simulink model "Model_14Bus_AC_DC_Microgrid"  (R2025a)
settings: Solver=ode23tb  StartTime=0.0  StopTime=0.1  MaxStep=1e-2  RelTol=1e-3
InitFcn:
  | Set_parameters_R2018
StopFcn:
  | Save_Data;
  | Graphics;
undefined symbols (not defined in the file): Clink, D1, Delta, dis1, dis10, dis11, dis12, dis13, dis14, dis2, dis3, dis4, dis5, dis6, dis7, dis8, dis9, Fc, Fnom, Hydride, Increment_MPPT, Ion, Ki_Ireg, Ki_VDCreg, Kp_Ireg, Kp_VDCreg, LimitL_Ireg, LimitL_VDCreg, Limits_MPPT, LimitU_Ireg, LimitU_VDCreg, Lithium, max_min, Metal, Nickel, P_Load_2, P_Load_3, Pnom, Pnom_T1, Pnom_T2, Pnom_T3, Pnom_xfo, Ql_Load_2, Ql_Load_3, R_Load_9, R_Load_DC, RL, Rl, RLff, Rls, sigbuilder_block, Ts, Ts_Control, Ts_Power, V1_LL_T3, Vf, Vfd, Vnom_dc, Vnom_DC, Vnom_Diesel ... (+5)
libraries: spsRMSLib x87, spsCurrentMeasurementLib x47, spsThreePhaseVIMeasurementLib x23, spsVoltageMeasurementLib x21, spsPowerLib x21, spsTHDLib x20, spsThreePhaseSeriesRLCBranchLib x20, spsSeriesRLCBranchLib x19, spsIGBTDiodeLib x14, spsThreePhaseBreakerLib x14, powerlib_extras x14, simulink x12
(part 8 of 9)

== system Model_14Bus_AC_DC_Microgrid/Bus_6 /PLL/Pll2 ==
  note: error
  note: d'
  note: Fundamental
  note: fase
      | total
  note: fase de la señal
  note: adelanta 90
  note: Este PLL calcula la fase respecto a una onda coseno
  señal : Inport
  w : Inport  Port=2
  Gain : Gain  Gain=-1  SaturateOnIntegerOverflow=on  OutDataTypeStr=Inherit: Same as input  ParamDataTypeStr=Inherit: Same as input
  Integrator : Integrator  InitialCondition=2*pi*60
  Integrator1 : Integrator  InitialCondition=2*pi*60
  Integrator2 : Integrator
  K : Gain  Gain=100  SaturateOnIntegerOverflow=on  OutDataTypeStr=Inherit: Same as input  ParamDataTypeStr=Inherit: Same as input
  Kp : Gain  Gain=10  SaturateOnIntegerOverflow=on  OutDataTypeStr=Inherit: Same as input  ParamDataTypeStr=Inherit: Same as input
  Kp1 : Gain  Gain=10  SaturateOnIntegerOverflow=on  OutDataTypeStr=Inherit: Same as input  ParamDataTypeStr=Inherit: Same as input
  Poduct : Product  SaturateOnIntegerOverflow=on  OutDataTypeStr=Inherit: Same as first input
  Poduct1 : Product  SaturateOnIntegerOverflow=on  OutDataTypeStr=Inherit: Same as first input
  Poduct2 : Product  SaturateOnIntegerOverflow=on  OutDataTypeStr=Inherit: Same as first input
  Sum : Sum  Inputs=|+-  SaturateOnIntegerOverflow=on
  Sum1 : Sum  SaturateOnIntegerOverflow=on
  Sum2 : Sum  Inputs=|-+  SaturateOnIntegerOverflow=on
  Trigonometric Function : Trigonometry
  Trigonometric Function1 : Trigonometry  Operator=cos
  f cos (rad) : Outport  VectorParamsAs1DForOutWhenUnconnected=off
  wires:
  Sum/1 -> Poduct/1, Poduct1/1
  Poduct/1 -> Kp/1
  Kp/1 -> Kp1/1
  Poduct2/1 -> Sum/2
  Trigonometric Function1/1 -> Poduct1/2, Poduct2/1
  Poduct1/1 -> K/1
  K/1 -> Integrator2/1
  Integrator2/1 -> Poduct2/2
  Integrator/1 -> Trigonometric Function/1, Sum2/2, Trigonometric Function1/1
  Integrator1/1 -> Sum2/1
  Sum2/1 -> f cos (rad)/1
  w/1 -> Sum1/1, Integrator1/1
  Kp1/1 -> Sum1/2
  Sum1/1 -> Integrator/1
  Trigonometric Function/1 -> Gain/1
  Gain/1 -> Poduct/2
  señal/1 -> Sum/1

== system Model_14Bus_AC_DC_Microgrid/Bus_6 /PLL/Pll3 ==
  note: error
  note: d'
  note: Fundamental
  note: fase
      | total
  note: fase de la señal
  note: adelanta 90
  note: Este PLL calcula la fase respecto a una onda coseno
  señal : Inport
  w : Inport  Port=2
  Gain : Gain  Gain=-1  SaturateOnIntegerOverflow=on  OutDataTypeStr=Inherit: Same as input  ParamDataTypeStr=Inherit: Same as input
  Integrator : Integrator  InitialCondition=2*pi*60
  Integrator1 : Integrator  InitialCondition=2*pi*60
  Integrator2 : Integrator
  K : Gain  Gain=100  SaturateOnIntegerOverflow=on  OutDataTypeStr=Inherit: Same as input  ParamDataTypeStr=Inherit: Same as input
  Kp : Gain  Gain=10  SaturateOnIntegerOverflow=on  OutDataTypeStr=Inherit: Same as input  ParamDataTypeStr=Inherit: Same as input
  Kp1 : Gain  Gain=10  SaturateOnIntegerOverflow=on  OutDataTypeStr=Inherit: Same as input  ParamDataTypeStr=Inherit: Same as input
  Poduct : Product  SaturateOnIntegerOverflow=on  OutDataTypeStr=Inherit: Same as first input
  Poduct1 : Product  SaturateOnIntegerOverflow=on  OutDataTypeStr=Inherit: Same as first input
  Poduct2 : Product  SaturateOnIntegerOverflow=on  OutDataTypeStr=Inherit: Same as first input
  Sum : Sum  Inputs=|+-  SaturateOnIntegerOverflow=on
  Sum1 : Sum  SaturateOnIntegerOverflow=on
  Sum2 : Sum  Inputs=|-+  SaturateOnIntegerOverflow=on
  Trigonometric Function : Trigonometry
  Trigonometric Function1 : Trigonometry  Operator=cos
  f cos (rad) : Outport  VectorParamsAs1DForOutWhenUnconnected=off
  wires:
  Sum/1 -> Poduct/1, Poduct1/1
  Poduct/1 -> Kp/1
  Kp/1 -> Kp1/1
  Poduct2/1 -> Sum/2
  Trigonometric Function1/1 -> Poduct1/2, Poduct2/1
  Poduct1/1 -> K/1
  K/1 -> Integrator2/1
  Integrator2/1 -> Poduct2/2
  Integrator/1 -> Trigonometric Function/1, Sum2/2, Trigonometric Function1/1
  Integrator1/1 -> Sum2/1
  Sum2/1 -> f cos (rad)/1
  w/1 -> Sum1/1, Integrator1/1
  Kp1/1 -> Sum1/2
  Sum1/1 -> Integrator/1
  Trigonometric Function/1 -> Gain/1
  Gain/1 -> Poduct/2
  señal/1 -> Sum/1

== system Model_14Bus_AC_DC_Microgrid/Bus_7/PLL/Pll1 ==
  note: error
  note: d'
  note: Fundamental
  note: fase
      | total
  note: fase de la señal
  note: adelanta 90
  note: Este PLL calcula la fase respecto a una onda coseno
  señal : Inport
  w : Inport  Port=2
  Gain : Gain  Gain=-1  SaturateOnIntegerOverflow=on  OutDataTypeStr=Inherit: Same as input  ParamDataTypeStr=Inherit: Same as input
  Integrator : Integrator  InitialCondition=2*pi*60
  Integrator1 : Integrator  InitialCondition=2*pi*60
  Integrator2 : Integrator
  K : Gain  Gain=100  SaturateOnIntegerOverflow=on  OutDataTypeStr=Inherit: Same as input  ParamDataTypeStr=Inherit: Same as input
  Kp : Gain  Gain=10  SaturateOnIntegerOverflow=on  OutDataTypeStr=Inherit: Same as input  ParamDataTypeStr=Inherit: Same as input
  Kp1 : Gain  Gain=10  SaturateOnIntegerOverflow=on  OutDataTypeStr=Inherit: Same as input  ParamDataTypeStr=Inherit: Same as input
  Poduct : Product  SaturateOnIntegerOverflow=on  OutDataTypeStr=Inherit: Same as first input
  Poduct1 : Product  SaturateOnIntegerOverflow=on  OutDataTypeStr=Inherit: Same as first input
  Poduct2 : Product  SaturateOnIntegerOverflow=on  OutDataTypeStr=Inherit: Same as first input
  Sum : Sum  Inputs=|+-  SaturateOnIntegerOverflow=on
  Sum1 : Sum  SaturateOnIntegerOverflow=on
  Sum2 : Sum  Inputs=|-+  SaturateOnIntegerOverflow=on
  Trigonometric Function : Trigonometry
  Trigonometric Function1 : Trigonometry  Operator=cos
  f cos (rad) : Outport  VectorParamsAs1DForOutWhenUnconnected=off
  wires:
  Sum/1 -> Poduct/1, Poduct1/1
  Poduct/1 -> Kp/1
  Kp/1 -> Kp1/1
  Poduct2/1 -> Sum/2
  Trigonometric Function1/1 -> Poduct1/2, Poduct2/1
  Poduct1/1 -> K/1
  K/1 -> Integrator2/1
  Integrator2/1 -> Poduct2/2
  Integrator/1 -> Trigonometric Function/1, Sum2/2, Trigonometric Function1/1
  Integrator1/1 -> Sum2/1
  Sum2/1 -> f cos (rad)/1
  w/1 -> Sum1/1, Integrator1/1
  Kp1/1 -> Sum1/2
  Sum1/1 -> Integrator/1
  Trigonometric Function/1 -> Gain/1
  Gain/1 -> Poduct/2
  señal/1 -> Sum/1

== system Model_14Bus_AC_DC_Microgrid/Bus_7/PLL/Pll2 ==
  note: error
  note: d'
  note: Fundamental
  note: fase
      | total
  note: fase de la señal
  note: adelanta 90
  note: Este PLL calcula la fase respecto a una onda coseno
  señal : Inport
  w : Inport  Port=2
  Gain : Gain  Gain=-1  SaturateOnIntegerOverflow=on  OutDataTypeStr=Inherit: Same as input  ParamDataTypeStr=Inherit: Same as input
  Integrator : Integrator  InitialCondition=2*pi*60
  Integrator1 : Integrator  InitialCondition=2*pi*60
  Integrator2 : Integrator
  K : Gain  Gain=100  SaturateOnIntegerOverflow=on  OutDataTypeStr=Inherit: Same as input  ParamDataTypeStr=Inherit: Same as input
  Kp : Gain  Gain=10  SaturateOnIntegerOverflow=on  OutDataTypeStr=Inherit: Same as input  ParamDataTypeStr=Inherit: Same as input
  Kp1 : Gain  Gain=10  SaturateOnIntegerOverflow=on  OutDataTypeStr=Inherit: Same as input  ParamDataTypeStr=Inherit: Same as input
  Poduct : Product  SaturateOnIntegerOverflow=on  OutDataTypeStr=Inherit: Same as first input
  Poduct1 : Product  SaturateOnIntegerOverflow=on  OutDataTypeStr=Inherit: Same as first input
  Poduct2 : Product  SaturateOnIntegerOverflow=on  OutDataTypeStr=Inherit: Same as first input
  Sum : Sum  Inputs=|+-  SaturateOnIntegerOverflow=on
  Sum1 : Sum  SaturateOnIntegerOverflow=on
  Sum2 : Sum  Inputs=|-+  SaturateOnIntegerOverflow=on
  Trigonometric Function : Trigonometry
  Trigonometric Function1 : Trigonometry  Operator=cos
  f cos (rad) : Outport  VectorParamsAs1DForOutWhenUnconnected=off
  wires:
  Sum/1 -> Poduct/1, Poduct1/1
  Poduct/1 -> Kp/1
  Kp/1 -> Kp1/1
  Poduct2/1 -> Sum/2
  Trigonometric Function1/1 -> Poduct1/2, Poduct2/1
  Poduct1/1 -> K/1
  K/1 -> Integrator2/1
  Integrator2/1 -> Poduct2/2
  Integrator/1 -> Trigonometric Function/1, Sum2/2, Trigonometric Function1/1
  Integrator1/1 -> Sum2/1
  Sum2/1 -> f cos (rad)/1
  w/1 -> Sum1/1, Integrator1/1
  Kp1/1 -> Sum1/2
  Sum1/1 -> Integrator/1
  Trigonometric Function/1 -> Gain/1
  Gain/1 -> Poduct/2
  señal/1 -> Sum/1

== system Model_14Bus_AC_DC_Microgrid/Bus_7/PLL/Pll3 ==
  note: error
  note: d'
  note: Fundamental
  note: fase
      | total
  note: fase de la señal
  note: adelanta 90
  note: Este PLL calcula la fase respecto a una onda coseno
  señal : Inport
  w : Inport  Port=2
  Gain : Gain  Gain=-1  SaturateOnIntegerOverflow=on  OutDataTypeStr=Inherit: Same as input  ParamDataTypeStr=Inherit: Same as input
  Integrator : Integrator  InitialCondition=2*pi*60
  Integrator1 : Integrator  InitialCondition=2*pi*60
  Integrator2 : Integrator
  K : Gain  Gain=100  SaturateOnIntegerOverflow=on  OutDataTypeStr=Inherit: Same as input  ParamDataTypeStr=Inherit: Same as input
  Kp : Gain  Gain=10  SaturateOnIntegerOverflow=on  OutDataTypeStr=Inherit: Same as input  ParamDataTypeStr=Inherit: Same as input
  Kp1 : Gain  Gain=10  SaturateOnIntegerOverflow=on  OutDataTypeStr=Inherit: Same as input  ParamDataTypeStr=Inherit: Same as input
  Poduct : Product  SaturateOnIntegerOverflow=on  OutDataTypeStr=Inherit: Same as first input
  Poduct1 : Product  SaturateOnIntegerOverflow=on  OutDataTypeStr=Inherit: Same as first input
  Poduct2 : Product  SaturateOnIntegerOverflow=on  OutDataTypeStr=Inherit: Same as first input
  Sum : Sum  Inputs=|+-  SaturateOnIntegerOverflow=on
  Sum1 : Sum  SaturateOnIntegerOverflow=on
  Sum2 : Sum  Inputs=|-+  SaturateOnIntegerOverflow=on
  Trigonometric Function : Trigonometry
  Trigonometric Function1 : Trigonometry  Operator=cos
  f cos (rad) : Outport  VectorParamsAs1DForOutWhenUnconnected=off
  wires:
  Sum/1 -> Poduct/1, Poduct1/1
  Poduct/1 -> Kp/1
  Kp/1 -> Kp1/1
  Poduct2/1 -> Sum/2
  Trigonometric Function1/1 -> Poduct1/2, Poduct2/1
  Poduct1/1 -> K/1
  K/1 -> Integrator2/1
  Integrator2/1 -> Poduct2/2
  Integrator/1 -> Trigonometric Function/1, Sum2/2, Trigonometric Function1/1
  Integrator1/1 -> Sum2/1
  Sum2/1 -> f cos (rad)/1
  w/1 -> Sum1/1, Integrator1/1
  Kp1/1 -> Sum1/2
  Sum1/1 -> Integrator/1
  Trigonometric Function/1 -> Gain/1
  Gain/1 -> Poduct/2
  señal/1 -> Sum/1

== system Model_14Bus_AC_DC_Microgrid/Bus_8      /PLL/Pll1 ==
  note: error
  note: d'
  note: Fundamental
  note: fase
      | total
  note: fase de la señal
  note: adelanta 90
  note: Este PLL calcula la fase respecto a una onda coseno
  señal : Inport
  w : Inport  Port=2
  Gain : Gain  Gain=-1  SaturateOnIntegerOverflow=on  OutDataTypeStr=Inherit: Same as input  ParamDataTypeStr=Inherit: Same as input
  Integrator : Integrator  InitialCondition=2*pi*60
  Integrator1 : Integrator  InitialCondition=2*pi*60
  Integrator2 : Integrator
  K : Gain  Gain=100  SaturateOnIntegerOverflow=on  OutDataTypeStr=Inherit: Same as input  ParamDataTypeStr=Inherit: Same as input
  Kp : Gain  Gain=10  SaturateOnIntegerOverflow=on  OutDataTypeStr=Inherit: Same as input  ParamDataTypeStr=Inherit: Same as input
  Kp1 : Gain  Gain=10  SaturateOnIntegerOverflow=on  OutDataTypeStr=Inherit: Same as input  ParamDataTypeStr=Inherit: Same as input
  Poduct : Product  SaturateOnIntegerOverflow=on  OutDataTypeStr=Inherit: Same as first input
  Poduct1 : Product  SaturateOnIntegerOverflow=on  OutDataTypeStr=Inherit: Same as first input
  Poduct2 : Product  SaturateOnIntegerOverflow=on  OutDataTypeStr=Inherit: Same as first input
  Sum : Sum  Inputs=|+-  SaturateOnIntegerOverflow=on
  Sum1 : Sum  SaturateOnIntegerOverflow=on
  Sum2 : Sum  Inputs=|-+  SaturateOnIntegerOverflow=on
  Trigonometric Function : Trigonometry
  Trigonometric Function1 : Trigonometry  Operator=cos
  f cos (rad) : Outport  VectorParamsAs1DForOutWhenUnconnected=off
  wires:
  Sum/1 -> Poduct/1, Poduct1/1
  Poduct/1 -> Kp/1
  Kp/1 -> Kp1/1
  Poduct2/1 -> Sum/2
  Trigonometric Function1/1 -> Poduct1/2, Poduct2/1
  Poduct1/1 -> K/1
  K/1 -> Integrator2/1
  Integrator2/1 -> Poduct2/2
  Integrator/1 -> Trigonometric Function/1, Sum2/2, Trigonometric Function1/1
  Integrator1/1 -> Sum2/1
  Sum2/1 -> f cos (rad)/1
  w/1 -> Sum1/1, Integrator1/1
  Kp1/1 -> Sum1/2
  Sum1/1 -> Integrator/1
  Trigonometric Function/1 -> Gain/1
  Gain/1 -> Poduct/2
  señal/1 -> Sum/1

== system Model_14Bus_AC_DC_Microgrid/Bus_8      /PLL/Pll2 ==
  note: error
  note: d'
  note: Fundamental
  note: fase
      | total
  note: fase de la señal
  note: adelanta 90
  note: Este PLL calcula la fase respecto a una onda coseno
  señal : Inport
  w : Inport  Port=2
  Gain : Gain  Gain=-1  SaturateOnIntegerOverflow=on  OutDataTypeStr=Inherit: Same as input  ParamDataTypeStr=Inherit: Same as input
  Integrator : Integrator  InitialCondition=2*pi*60
  Integrator1 : Integrator  InitialCondition=2*pi*60
  Integrator2 : Integrator
  K : Gain  Gain=100  SaturateOnIntegerOverflow=on  OutDataTypeStr=Inherit: Same as input  ParamDataTypeStr=Inherit: Same as input
  Kp : Gain  Gain=10  SaturateOnIntegerOverflow=on  OutDataTypeStr=Inherit: Same as input  ParamDataTypeStr=Inherit: Same as input
  Kp1 : Gain  Gain=10  SaturateOnIntegerOverflow=on  OutDataTypeStr=Inherit: Same as input  ParamDataTypeStr=Inherit: Same as input
  Poduct : Product  SaturateOnIntegerOverflow=on  OutDataTypeStr=Inherit: Same as first input
  Poduct1 : Product  SaturateOnIntegerOverflow=on  OutDataTypeStr=Inherit: Same as first input
  Poduct2 : Product  SaturateOnIntegerOverflow=on  OutDataTypeStr=Inherit: Same as first input
  Sum : Sum  Inputs=|+-  SaturateOnIntegerOverflow=on
  Sum1 : Sum  SaturateOnIntegerOverflow=on
  Sum2 : Sum  Inputs=|-+  SaturateOnIntegerOverflow=on
  Trigonometric Function : Trigonometry
  Trigonometric Function1 : Trigonometry  Operator=cos
  f cos (rad) : Outport  VectorParamsAs1DForOutWhenUnconnected=off
  wires:
  Sum/1 -> Poduct/1, Poduct1/1
  Poduct/1 -> Kp/1
  Kp/1 -> Kp1/1
  Poduct2/1 -> Sum/2
  Trigonometric Function1/1 -> Poduct1/2, Poduct2/1
  Poduct1/1 -> K/1
  K/1 -> Integrator2/1
  Integrator2/1 -> Poduct2/2
  Integrator/1 -> Trigonometric Function/1, Sum2/2, Trigonometric Function1/1
  Integrator1/1 -> Sum2/1
  Sum2/1 -> f cos (rad)/1
  w/1 -> Sum1/1, Integrator1/1
  Kp1/1 -> Sum1/2
  Sum1/1 -> Integrator/1
  Trigonometric Function/1 -> Gain/1
  Gain/1 -> Poduct/2
  señal/1 -> Sum/1

== system Model_14Bus_AC_DC_Microgrid/Bus_8      /PLL/Pll3 ==
  note: error
  note: d'
  note: Fundamental
  note: fase
      | total
  note: fase de la señal
  note: adelanta 90
  note: Este PLL calcula la fase respecto a una onda coseno
  señal : Inport
  w : Inport  Port=2
  Gain : Gain  Gain=-1  SaturateOnIntegerOverflow=on  OutDataTypeStr=Inherit: Same as input  ParamDataTypeStr=Inherit: Same as input
  Integrator : Integrator  InitialCondition=2*pi*60
  Integrator1 : Integrator  InitialCondition=2*pi*60
  Integrator2 : Integrator
  K : Gain  Gain=100  SaturateOnIntegerOverflow=on  OutDataTypeStr=Inherit: Same as input  ParamDataTypeStr=Inherit: Same as input
  Kp : Gain  Gain=10  SaturateOnIntegerOverflow=on  OutDataTypeStr=Inherit: Same as input  ParamDataTypeStr=Inherit: Same as input
  Kp1 : Gain  Gain=10  SaturateOnIntegerOverflow=on  OutDataTypeStr=Inherit: Same as input  ParamDataTypeStr=Inherit: Same as input
  Poduct : Product  SaturateOnIntegerOverflow=on  OutDataTypeStr=Inherit: Same as first input
  Poduct1 : Product  SaturateOnIntegerOverflow=on  OutDataTypeStr=Inherit: Same as first input
  Poduct2 : Product  SaturateOnIntegerOverflow=on  OutDataTypeStr=Inherit: Same as first input
  Sum : Sum  Inputs=|+-  SaturateOnIntegerOverflow=on
  Sum1 : Sum  SaturateOnIntegerOverflow=on
  Sum2 : Sum  Inputs=|-+  SaturateOnIntegerOverflow=on
  Trigonometric Function : Trigonometry
  Trigonometric Function1 : Trigonometry  Operator=cos
  f cos (rad) : Outport  VectorParamsAs1DForOutWhenUnconnected=off
  wires:
  Sum/1 -> Poduct/1, Poduct1/1
  Poduct/1 -> Kp/1
  Kp/1 -> Kp1/1
  Poduct2/1 -> Sum/2
  Trigonometric Function1/1 -> Poduct1/2, Poduct2/1
  Poduct1/1 -> K/1
  K/1 -> Integrator2/1
  Integrator2/1 -> Poduct2/2
  Integrator/1 -> Trigonometric Function/1, Sum2/2, Trigonometric Function1/1
  Integrator1/1 -> Sum2/1
  Sum2/1 -> f cos (rad)/1
  w/1 -> Sum1/1, Integrator1/1
  Kp1/1 -> Sum1/2
  Sum1/1 -> Integrator/1
  Trigonometric Function/1 -> Gain/1
  Gain/1 -> Poduct/2
  señal/1 -> Sum/1

== system Model_14Bus_AC_DC_Microgrid/Bus_9/PLL/Pll1 ==
  note: error
  note: d'
  note: Fundamental
  note: fase
      | total
  note: fase de la señal
  note: adelanta 90
  note: Este PLL calcula la fase respecto a una onda coseno
  señal : Inport
  w : Inport  Port=2
  Gain : Gain  Gain=-1  SaturateOnIntegerOverflow=on  OutDataTypeStr=Inherit: Same as input  ParamDataTypeStr=Inherit: Same as input
  Integrator : Integrator  InitialCondition=2*pi*60
  Integrator1 : Integrator  InitialCondition=2*pi*60
  Integrator2 : Integrator
  K : Gain  Gain=100  SaturateOnIntegerOverflow=on  OutDataTypeStr=Inherit: Same as input  ParamDataTypeStr=Inherit: Same as input
  Kp : Gain  Gain=10  SaturateOnIntegerOverflow=on  OutDataTypeStr=Inherit: Same as input  ParamDataTypeStr=Inherit: Same as input
  Kp1 : Gain  Gain=10  SaturateOnIntegerOverflow=on  OutDataTypeStr=Inherit: Same as input  ParamDataTypeStr=Inherit: Same as input
  Poduct : Product  SaturateOnIntegerOverflow=on  OutDataTypeStr=Inherit: Same as first input
  Poduct1 : Product  SaturateOnIntegerOverflow=on  OutDataTypeStr=Inherit: Same as first input
  Poduct2 : Product  SaturateOnIntegerOverflow=on  OutDataTypeStr=Inherit: Same as first input
  Sum : Sum  Inputs=|+-  SaturateOnIntegerOverflow=on
  Sum1 : Sum  SaturateOnIntegerOverflow=on
  Sum2 : Sum  Inputs=|-+  SaturateOnIntegerOverflow=on
  Trigonometric Function : Trigonometry
  Trigonometric Function1 : Trigonometry  Operator=cos
  f cos (rad) : Outport  VectorParamsAs1DForOutWhenUnconnected=off
  wires:
  Sum/1 -> Poduct/1, Poduct1/1
  Poduct/1 -> Kp/1
  Kp/1 -> Kp1/1
  Poduct2/1 -> Sum/2
  Trigonometric Function1/1 -> Poduct1/2, Poduct2/1
  Poduct1/1 -> K/1
  K/1 -> Integrator2/1
  Integrator2/1 -> Poduct2/2
  Integrator/1 -> Trigonometric Function/1, Sum2/2, Trigonometric Function1/1
  Integrator1/1 -> Sum2/1
  Sum2/1 -> f cos (rad)/1
  w/1 -> Sum1/1, Integrator1/1
  Kp1/1 -> Sum1/2
  Sum1/1 -> Integrator/1
  Trigonometric Function/1 -> Gain/1
  Gain/1 -> Poduct/2
  señal/1 -> Sum/1

== system Model_14Bus_AC_DC_Microgrid/Bus_9/PLL/Pll2 ==
  note: error
  note: d'
  note: Fundamental
  note: fase
      | total
  note: fase de la señal
  note: adelanta 90
  note: Este PLL calcula la fase respecto a una onda coseno
  señal : Inport
  w : Inport  Port=2
  Gain : Gain  Gain=-1  SaturateOnIntegerOverflow=on  OutDataTypeStr=Inherit: Same as input  ParamDataTypeStr=Inherit: Same as input
  Integrator : Integrator  InitialCondition=2*pi*60
  Integrator1 : Integrator  InitialCondition=2*pi*60
  Integrator2 : Integrator
  K : Gain  Gain=100  SaturateOnIntegerOverflow=on  OutDataTypeStr=Inherit: Same as input  ParamDataTypeStr=Inherit: Same as input
  Kp : Gain  Gain=10  SaturateOnIntegerOverflow=on  OutDataTypeStr=Inherit: Same as input  ParamDataTypeStr=Inherit: Same as input
  Kp1 : Gain  Gain=10  SaturateOnIntegerOverflow=on  OutDataTypeStr=Inherit: Same as input  ParamDataTypeStr=Inherit: Same as input
  Poduct : Product  SaturateOnIntegerOverflow=on  OutDataTypeStr=Inherit: Same as first input
  Poduct1 : Product  SaturateOnIntegerOverflow=on  OutDataTypeStr=Inherit: Same as first input
  Poduct2 : Product  SaturateOnIntegerOverflow=on  OutDataTypeStr=Inherit: Same as first input
  Sum : Sum  Inputs=|+-  SaturateOnIntegerOverflow=on
  Sum1 : Sum  SaturateOnIntegerOverflow=on
  Sum2 : Sum  Inputs=|-+  SaturateOnIntegerOverflow=on
  Trigonometric Function : Trigonometry
  Trigonometric Function1 : Trigonometry  Operator=cos
  f cos (rad) : Outport  VectorParamsAs1DForOutWhenUnconnected=off
  wires:
  Sum/1 -> Poduct/1, Poduct1/1
  Poduct/1 -> Kp/1
  Kp/1 -> Kp1/1
  Poduct2/1 -> Sum/2
  Trigonometric Function1/1 -> Poduct1/2, Poduct2/1
  Poduct1/1 -> K/1
  K/1 -> Integrator2/1
  Integrator2/1 -> Poduct2/2
  Integrator/1 -> Trigonometric Function/1, Sum2/2, Trigonometric Function1/1
  Integrator1/1 -> Sum2/1
  Sum2/1 -> f cos (rad)/1
  w/1 -> Sum1/1, Integrator1/1
  Kp1/1 -> Sum1/2
  Sum1/1 -> Integrator/1
  Trigonometric Function/1 -> Gain/1
  Gain/1 -> Poduct/2
  señal/1 -> Sum/1

== system Model_14Bus_AC_DC_Microgrid/Bus_9/PLL/Pll3 ==
  note: error
  note: d'
  note: Fundamental
  note: fase
      | total
  note: fase de la señal
  note: adelanta 90
  note: Este PLL calcula la fase respecto a una onda coseno
  señal : Inport
  w : Inport  Port=2
  Gain : Gain  Gain=-1  SaturateOnIntegerOverflow=on  OutDataTypeStr=Inherit: Same as input  ParamDataTypeStr=Inherit: Same as input
  Integrator : Integrator  InitialCondition=2*pi*60
  Integrator1 : Integrator  InitialCondition=2*pi*60
  Integrator2 : Integrator
  K : Gain  Gain=100  SaturateOnIntegerOverflow=on  OutDataTypeStr=Inherit: Same as input  ParamDataTypeStr=Inherit: Same as input
  Kp : Gain  Gain=10  SaturateOnIntegerOverflow=on  OutDataTypeStr=Inherit: Same as input  ParamDataTypeStr=Inherit: Same as input
  Kp1 : Gain  Gain=10  SaturateOnIntegerOverflow=on  OutDataTypeStr=Inherit: Same as input  ParamDataTypeStr=Inherit: Same as input
  Poduct : Product  SaturateOnIntegerOverflow=on  OutDataTypeStr=Inherit: Same as first input
  Poduct1 : Product  SaturateOnIntegerOverflow=on  OutDataTypeStr=Inherit: Same as first input
  Poduct2 : Product  SaturateOnIntegerOverflow=on  OutDataTypeStr=Inherit: Same as first input
  Sum : Sum  Inputs=|+-  SaturateOnIntegerOverflow=on
  Sum1 : Sum  SaturateOnIntegerOverflow=on
  Sum2 : Sum  Inputs=|-+  SaturateOnIntegerOverflow=on
  Trigonometric Function : Trigonometry
  Trigonometric Function1 : Trigonometry  Operator=cos
  f cos (rad) : Outport  VectorParamsAs1DForOutWhenUnconnected=off
  wires:
  Sum/1 -> Poduct/1, Poduct1/1
  Poduct/1 -> Kp/1
  Kp/1 -> Kp1/1
  Poduct2/1 -> Sum/2
  Trigonometric Function1/1 -> Poduct1/2, Poduct2/1
  Poduct1/1 -> K/1
  K/1 -> Integrator2/1
  Integrator2/1 -> Poduct2/2
  Integrator/1 -> Trigonometric Function/1, Sum2/2, Trigonometric Function1/1
  Integrator1/1 -> Sum2/1
  Sum2/1 -> f cos (rad)/1
  w/1 -> Sum1/1, Integrator1/1
  Kp1/1 -> Sum1/2
  Sum1/1 -> Integrator/1
  Trigonometric Function/1 -> Gain/1
  Gain/1 -> Poduct/2
  señal/1 -> Sum/1

== system Model_14Bus_AC_DC_Microgrid/Bus_AC PV /PLL/Pll1 ==
  note: error
  note: d'
  note: Fundamental
  note: fase
      | total
  note: fase de la señal
  note: adelanta 90
  note: Este PLL calcula la fase respecto a una onda coseno
  señal : Inport
  w : Inport  Port=2
  Gain : Gain  Gain=-1  SaturateOnIntegerOverflow=on  OutDataTypeStr=Inherit: Same as input  ParamDataTypeStr=Inherit: Same as input
  Integrator : Integrator  InitialCondition=2*pi*60
  Integrator1 : Integrator  InitialCondition=2*pi*60
  Integrator2 : Integrator
  K : Gain  Gain=100  SaturateOnIntegerOverflow=on  OutDataTypeStr=Inherit: Same as input  ParamDataTypeStr=Inherit: Same as input
  Kp : Gain  Gain=10  SaturateOnIntegerOverflow=on  OutDataTypeStr=Inherit: Same as input  ParamDataTypeStr=Inherit: Same as input
  Kp1 : Gain  Gain=10  SaturateOnIntegerOverflow=on  OutDataTypeStr=Inherit: Same as input  ParamDataTypeStr=Inherit: Same as input
  Poduct : Product  SaturateOnIntegerOverflow=on  OutDataTypeStr=Inherit: Same as first input
  Poduct1 : Product  SaturateOnIntegerOverflow=on  OutDataTypeStr=Inherit: Same as first input
  Poduct2 : Product  SaturateOnIntegerOverflow=on  OutDataTypeStr=Inherit: Same as first input
  Sum : Sum  Inputs=|+-  SaturateOnIntegerOverflow=on
  Sum1 : Sum  SaturateOnIntegerOverflow=on
  Sum2 : Sum  Inputs=|-+  SaturateOnIntegerOverflow=on
  Trigonometric Function : Trigonometry
  Trigonometric Function1 : Trigonometry  Operator=cos
  f cos (rad) : Outport  VectorParamsAs1DForOutWhenUnconnected=off
  wires:
  Sum/1 -> Poduct/1, Poduct1/1
  Poduct/1 -> Kp/1
  Kp/1 -> Kp1/1
  Poduct2/1 -> Sum/2
  Trigonometric Function1/1 -> Poduct1/2, Poduct2/1
  Poduct1/1 -> K/1
  K/1 -> Integrator2/1
  Integrator2/1 -> Poduct2/2
  Integrator/1 -> Trigonometric Function/1, Sum2/2, Trigonometric Function1/1
  Integrator1/1 -> Sum2/1
  Sum2/1 -> f cos (rad)/1
  w/1 -> Sum1/1, Integrator1/1
  Kp1/1 -> Sum1/2
  Sum1/1 -> Integrator/1
  Trigonometric Function/1 -> Gain/1
  Gain/1 -> Poduct/2
  señal/1 -> Sum/1

== system Model_14Bus_AC_DC_Microgrid/Bus_AC PV /PLL/Pll2 ==
  note: error
  note: d'
  note: Fundamental
  note: fase
      | total
  note: fase de la señal
  note: adelanta 90
  note: Este PLL calcula la fase respecto a una onda coseno
  señal : Inport
  w : Inport  Port=2
  Gain : Gain  Gain=-1  SaturateOnIntegerOverflow=on  OutDataTypeStr=Inherit: Same as input  ParamDataTypeStr=Inherit: Same as input
  Integrator : Integrator  InitialCondition=2*pi*60
  Integrator1 : Integrator  InitialCondition=2*pi*60
  Integrator2 : Integrator
  K : Gain  Gain=100  SaturateOnIntegerOverflow=on  OutDataTypeStr=Inherit: Same as input  ParamDataTypeStr=Inherit: Same as input
  Kp : Gain  Gain=10  SaturateOnIntegerOverflow=on  OutDataTypeStr=Inherit: Same as input  ParamDataTypeStr=Inherit: Same as input
  Kp1 : Gain  Gain=10  SaturateOnIntegerOverflow=on  OutDataTypeStr=Inherit: Same as input  ParamDataTypeStr=Inherit: Same as input
  Poduct : Product  SaturateOnIntegerOverflow=on  OutDataTypeStr=Inherit: Same as first input
  Poduct1 : Product  SaturateOnIntegerOverflow=on  OutDataTypeStr=Inherit: Same as first input
  Poduct2 : Product  SaturateOnIntegerOverflow=on  OutDataTypeStr=Inherit: Same as first input
  Sum : Sum  Inputs=|+-  SaturateOnIntegerOverflow=on
  Sum1 : Sum  SaturateOnIntegerOverflow=on
  Sum2 : Sum  Inputs=|-+  SaturateOnIntegerOverflow=on
  Trigonometric Function : Trigonometry
  Trigonometric Function1 : Trigonometry  Operator=cos
  f cos (rad) : Outport  VectorParamsAs1DForOutWhenUnconnected=off
  wires:
  Sum/1 -> Poduct/1, Poduct1/1
  Poduct/1 -> Kp/1
  Kp/1 -> Kp1/1
  Poduct2/1 -> Sum/2
  Trigonometric Function1/1 -> Poduct1/2, Poduct2/1
  Poduct1/1 -> K/1
  K/1 -> Integrator2/1
  Integrator2/1 -> Poduct2/2
  Integrator/1 -> Trigonometric Function/1, Sum2/2, Trigonometric Function1/1
  Integrator1/1 -> Sum2/1
  Sum2/1 -> f cos (rad)/1
  w/1 -> Sum1/1, Integrator1/1
  Kp1/1 -> Sum1/2
  Sum1/1 -> Integrator/1
  Trigonometric Function/1 -> Gain/1
  Gain/1 -> Poduct/2
  señal/1 -> Sum/1

== system Model_14Bus_AC_DC_Microgrid/Bus_AC PV /PLL/Pll3 ==
  note: error
  note: d'
  note: Fundamental
  note: fase
      | total
  note: fase de la señal
  note: adelanta 90
  note: Este PLL calcula la fase respecto a una onda coseno
  señal : Inport
  w : Inport  Port=2
  Gain : Gain  Gain=-1  SaturateOnIntegerOverflow=on  OutDataTypeStr=Inherit: Same as input  ParamDataTypeStr=Inherit: Same as input
  Integrator : Integrator  InitialCondition=2*pi*60
  Integrator1 : Integrator  InitialCondition=2*pi*60
  Integrator2 : Integrator
  K : Gain  Gain=100  SaturateOnIntegerOverflow=on  OutDataTypeStr=Inherit: Same as input  ParamDataTypeStr=Inherit: Same as input
  Kp : Gain  Gain=10  SaturateOnIntegerOverflow=on  OutDataTypeStr=Inherit: Same as input  ParamDataTypeStr=Inherit: Same as input
  Kp1 : Gain  Gain=10  SaturateOnIntegerOverflow=on  OutDataTypeStr=Inherit: Same as input  ParamDataTypeStr=Inherit: Same as input
  Poduct : Product  SaturateOnIntegerOverflow=on  OutDataTypeStr=Inherit: Same as first input
  Poduct1 : Product  SaturateOnIntegerOverflow=on  OutDataTypeStr=Inherit: Same as first input
  Poduct2 : Product  SaturateOnIntegerOverflow=on  OutDataTypeStr=Inherit: Same as first input
  Sum : Sum  Inputs=|+-  SaturateOnIntegerOverflow=on
  Sum1 : Sum  SaturateOnIntegerOverflow=on
  Sum2 : Sum  Inputs=|-+  SaturateOnIntegerOverflow=on
  Trigonometric Function : Trigonometry
  Trigonometric Function1 : Trigonometry  Operator=cos
  f cos (rad) : Outport  VectorParamsAs1DForOutWhenUnconnected=off
  wires:
  Sum/1 -> Poduct/1, Poduct1/1
  Poduct/1 -> Kp/1
  Kp/1 -> Kp1/1
  Poduct2/1 -> Sum/2
  Trigonometric Function1/1 -> Poduct1/2, Poduct2/1
  Poduct1/1 -> K/1
  K/1 -> Integrator2/1
  Integrator2/1 -> Poduct2/2
  Integrator/1 -> Trigonometric Function/1, Sum2/2, Trigonometric Function1/1
  Integrator1/1 -> Sum2/1
  Sum2/1 -> f cos (rad)/1
  w/1 -> Sum1/1, Integrator1/1
  Kp1/1 -> Sum1/2
  Sum1/1 -> Integrator/1
  Trigonometric Function/1 -> Gain/1
  Gain/1 -> Poduct/2
  señal/1 -> Sum/1

== system Model_14Bus_AC_DC_Microgrid/Bus_AC//DC3/Battery system/Ripple Calculations ==
  Signal : Inport
  Reset : Inport  Port=2
  0 : Constant  Value=2
  1 : Constant  Value=2
  Display10 : Display
  Display2 : Display
  Mean1 : spsMeanLib/Mean  Freq=10  Vinit=0  Ts=0
  MinMax Running Resettable : simulink/Math Operations/MinMax Running Resettable  Function=max  vinit=0.0
  MinMax Running Resettable1 : simulink/Math Operations/MinMax Running Resettable  Function=min  vinit=0.0
  Product : Product
  Product1 : Product
  Sum : Sum  Inputs=|+-
  Sum1 : Sum  Inputs=|-+
  Switch1 : Switch  Criteria=u2 > Threshold  SaturateOnIntegerOverflow=off  InputSameDT=off
  Switch2 : Switch  Criteria=u2 > Threshold  SaturateOnIntegerOverflow=off  InputSameDT=off
  Switch3 : Switch  Criteria=u2 > Threshold  SaturateOnIntegerOverflow=off  InputSameDT=off
  Ripple in Buck : Outport  VectorParamsAs1DForOutWhenUnconnected=off
  Ripple in Boost : Outport  Port=2  VectorParamsAs1DForOutWhenUnconnected=off
  wires:
  1/1 -> Product1/2
  [I_ref] -> Switch2/2, Switch3/2
  Product1/1 -> Switch3/3
  0/1 -> Product/2
  Switch2/1 -> Ripple in Buck/1
  Switch3/1 -> Ripple in Boost/1
  Product/1 -> Switch2/1
  Signal/1 -> Mean1/1, MinMax Running Resettable1/1, MinMax Running Resettable/1
  Switch1/1 -> Sum1/2, Sum/2
  MinMax Running Resettable/1 -> Sum/1, Display2/1
  MinMax Running Resettable1/1 -> Sum1/1, Display10/1
  Sum/1 -> Product/1
  Reset/1 -> Switch1/2, MinMax Running Resettable1/2, MinMax Running Resettable/2
  Sum1/1 -> Product1/1
  Mean1/1 -> Switch1/3

== system Model_14Bus_AC_DC_Microgrid/Bus_AC//DC3/PV system/Pmean ==
  Product : Product  RndMeth=Zero
  WkW : Gain  Gain=1/1000
  P : Outport  VectorParamsAs1DForOutWhenUnconnected=off
  V : Outport  Port=2  VectorParamsAs1DForOutWhenUnconnected=off
  wires:
  [Vmean_PV] -> Product/1, V/1
  Product/1 -> WkW/1
  [Imean_PV] -> Product/2
  WkW/1 -> P/1  "Pmean_PV (kW)"

== system Model_14Bus_AC_DC_Microgrid/Bus_AC//DC4/PLL/Pll1 ==
  note: error
  note: d'
  note: Fundamental
  note: fase
      | total
  note: fase de la señal
  note: adelanta 90
  note: Este PLL calcula la fase respecto a una onda coseno
  señal : Inport
  w : Inport  Port=2
  Gain : Gain  Gain=-1  SaturateOnIntegerOverflow=on  OutDataTypeStr=Inherit: Same as input  ParamDataTypeStr=Inherit: Same as input
  Integrator : Integrator  InitialCondition=2*pi*60
  Integrator1 : Integrator  InitialCondition=2*pi*60
  Integrator2 : Integrator
  K : Gain  Gain=100  SaturateOnIntegerOverflow=on  OutDataTypeStr=Inherit: Same as input  ParamDataTypeStr=Inherit: Same as input
  Kp : Gain  Gain=10  SaturateOnIntegerOverflow=on  OutDataTypeStr=Inherit: Same as input  ParamDataTypeStr=Inherit: Same as input
  Kp1 : Gain  Gain=10  SaturateOnIntegerOverflow=on  OutDataTypeStr=Inherit: Same as input  ParamDataTypeStr=Inherit: Same as input
  Poduct : Product  SaturateOnIntegerOverflow=on  OutDataTypeStr=Inherit: Same as first input
  Poduct1 : Product  SaturateOnIntegerOverflow=on  OutDataTypeStr=Inherit: Same as first input
  Poduct2 : Product  SaturateOnIntegerOverflow=on  OutDataTypeStr=Inherit: Same as first input
  Sum : Sum  Inputs=|+-  SaturateOnIntegerOverflow=on
  Sum1 : Sum  SaturateOnIntegerOverflow=on
  Sum2 : Sum  Inputs=|-+  SaturateOnIntegerOverflow=on
  Trigonometric Function : Trigonometry
  Trigonometric Function1 : Trigonometry  Operator=cos
  f cos (rad) : Outport  VectorParamsAs1DForOutWhenUnconnected=off
  wires:
  Sum/1 -> Poduct/1, Poduct1/1
  Poduct/1 -> Kp/1
  Kp/1 -> Kp1/1
  Poduct2/1 -> Sum/2
  Trigonometric Function1/1 -> Poduct1/2, Poduct2/1
  Poduct1/1 -> K/1
  K/1 -> Integrator2/1
  Integrator2/1 -> Poduct2/2
  Integrator/1 -> Trigonometric Function/1, Sum2/2, Trigonometric Function1/1
  Integrator1/1 -> Sum2/1
  Sum2/1 -> f cos (rad)/1
  w/1 -> Sum1/1, Integrator1/1
  Kp1/1 -> Sum1/2
  Sum1/1 -> Integrator/1
  Trigonometric Function/1 -> Gain/1
  Gain/1 -> Poduct/2
  señal/1 -> Sum/1

== system Model_14Bus_AC_DC_Microgrid/Bus_AC//DC4/PLL/Pll2 ==
  note: error
  note: d'
  note: Fundamental
  note: fase
      | total
  note: fase de la señal
  note: adelanta 90
  note: Este PLL calcula la fase respecto a una onda coseno
  señal : Inport
  w : Inport  Port=2
  Gain : Gain  Gain=-1  SaturateOnIntegerOverflow=on  OutDataTypeStr=Inherit: Same as input  ParamDataTypeStr=Inherit: Same as input
  Integrator : Integrator  InitialCondition=2*pi*60
  Integrator1 : Integrator  InitialCondition=2*pi*60
  Integrator2 : Integrator
  K : Gain  Gain=100  SaturateOnIntegerOverflow=on  OutDataTypeStr=Inherit: Same as input  ParamDataTypeStr=Inherit: Same as input
  Kp : Gain  Gain=10  SaturateOnIntegerOverflow=on  OutDataTypeStr=Inherit: Same as input  ParamDataTypeStr=Inherit: Same as input
  Kp1 : Gain  Gain=10  SaturateOnIntegerOverflow=on  OutDataTypeStr=Inherit: Same as input  ParamDataTypeStr=Inherit: Same as input
  Poduct : Product  SaturateOnIntegerOverflow=on  OutDataTypeStr=Inherit: Same as first input
  Poduct1 : Product  SaturateOnIntegerOverflow=on  OutDataTypeStr=Inherit: Same as first input
  Poduct2 : Product  SaturateOnIntegerOverflow=on  OutDataTypeStr=Inherit: Same as first input
  Sum : Sum  Inputs=|+-  SaturateOnIntegerOverflow=on
  Sum1 : Sum  SaturateOnIntegerOverflow=on
  Sum2 : Sum  Inputs=|-+  SaturateOnIntegerOverflow=on
  Trigonometric Function : Trigonometry
  Trigonometric Function1 : Trigonometry  Operator=cos
  f cos (rad) : Outport  VectorParamsAs1DForOutWhenUnconnected=off
  wires:
  Sum/1 -> Poduct/1, Poduct1/1
  Poduct/1 -> Kp/1
  Kp/1 -> Kp1/1
  Poduct2/1 -> Sum/2
  Trigonometric Function1/1 -> Poduct1/2, Poduct2/1
  Poduct1/1 -> K/1
  K/1 -> Integrator2/1
  Integrator2/1 -> Poduct2/2
  Integrator/1 -> Trigonometric Function/1, Sum2/2, Trigonometric Function1/1
  Integrator1/1 -> Sum2/1
  Sum2/1 -> f cos (rad)/1
  w/1 -> Sum1/1, Integrator1/1
  Kp1/1 -> Sum1/2
  Sum1/1 -> Integrator/1
  Trigonometric Function/1 -> Gain/1
  Gain/1 -> Poduct/2
  señal/1 -> Sum/1

== system Model_14Bus_AC_DC_Microgrid/Bus_AC//DC4/PLL/Pll3 ==
  note: error
  note: d'
  note: Fundamental
  note: fase
      | total
  note: fase de la señal
  note: adelanta 90
  note: Este PLL calcula la fase respecto a una onda coseno
  señal : Inport
  w : Inport  Port=2
  Gain : Gain  Gain=-1  SaturateOnIntegerOverflow=on  OutDataTypeStr=Inherit: Same as input  ParamDataTypeStr=Inherit: Same as input
  Integrator : Integrator  InitialCondition=2*pi*60
  Integrator1 : Integrator  InitialCondition=2*pi*60
  Integrator2 : Integrator
  K : Gain  Gain=100  SaturateOnIntegerOverflow=on  OutDataTypeStr=Inherit: Same as input  ParamDataTypeStr=Inherit: Same as input
  Kp : Gain  Gain=10  SaturateOnIntegerOverflow=on  OutDataTypeStr=Inherit: Same as input  ParamDataTypeStr=Inherit: Same as input
  Kp1 : Gain  Gain=10  SaturateOnIntegerOverflow=on  OutDataTypeStr=Inherit: Same as input  ParamDataTypeStr=Inherit: Same as input
  Poduct : Product  SaturateOnIntegerOverflow=on  OutDataTypeStr=Inherit: Same as first input
  Poduct1 : Product  SaturateOnIntegerOverflow=on  OutDataTypeStr=Inherit: Same as first input
  Poduct2 : Product  SaturateOnIntegerOverflow=on  OutDataTypeStr=Inherit: Same as first input
  Sum : Sum  Inputs=|+-  SaturateOnIntegerOverflow=on
  Sum1 : Sum  SaturateOnIntegerOverflow=on
  Sum2 : Sum  Inputs=|-+  SaturateOnIntegerOverflow=on
  Trigonometric Function : Trigonometry
  Trigonometric Function1 : Trigonometry  Operator=cos
  f cos (rad) : Outport  VectorParamsAs1DForOutWhenUnconnected=off
  wires:
  Sum/1 -> Poduct/1, Poduct1/1
  Poduct/1 -> Kp/1
  Kp/1 -> Kp1/1
  Poduct2/1 -> Sum/2
  Trigonometric Function1/1 -> Poduct1/2, Poduct2/1
  Poduct1/1 -> K/1
  K/1 -> Integrator2/1
  Integrator2/1 -> Poduct2/2
  Integrator/1 -> Trigonometric Function/1, Sum2/2, Trigonometric Function1/1
  Integrator1/1 -> Sum2/1
  Sum2/1 -> f cos (rad)/1
  w/1 -> Sum1/1, Integrator1/1
  Kp1/1 -> Sum1/2
  Sum1/1 -> Integrator/1
  Trigonometric Function/1 -> Gain/1
  Gain/1 -> Poduct/2
  señal/1 -> Sum/1

== system Model_14Bus_AC_DC_Microgrid/Bus_AC//DC5/PLL/Pll1 ==
  note: error
  note: d'
  note: Fundamental
  note: fase
      | total
  note: fase de la señal
  note: adelanta 90
  note: Este PLL calcula la fase respecto a una onda coseno
  señal : Inport
  w : Inport  Port=2
  Gain : Gain  Gain=-1  SaturateOnIntegerOverflow=on  OutDataTypeStr=Inherit: Same as input  ParamDataTypeStr=Inherit: Same as input
  Integrator : Integrator  InitialCondition=2*pi*60
  Integrator1 : Integrator  InitialCondition=2*pi*60
  Integrator2 : Integrator
  K : Gain  Gain=100  SaturateOnIntegerOverflow=on  OutDataTypeStr=Inherit: Same as input  ParamDataTypeStr=Inherit: Same as input
  Kp : Gain  Gain=10  SaturateOnIntegerOverflow=on  OutDataTypeStr=Inherit: Same as input  ParamDataTypeStr=Inherit: Same as input
  Kp1 : Gain  Gain=10  SaturateOnIntegerOverflow=on  OutDataTypeStr=Inherit: Same as input  ParamDataTypeStr=Inherit: Same as input
  Poduct : Product  SaturateOnIntegerOverflow=on  OutDataTypeStr=Inherit: Same as first input
  Poduct1 : Product  SaturateOnIntegerOverflow=on  OutDataTypeStr=Inherit: Same as first input
  Poduct2 : Product  SaturateOnIntegerOverflow=on  OutDataTypeStr=Inherit: Same as first input
  Sum : Sum  Inputs=|+-  SaturateOnIntegerOverflow=on
  Sum1 : Sum  SaturateOnIntegerOverflow=on
  Sum2 : Sum  Inputs=|-+  SaturateOnIntegerOverflow=on
  Trigonometric Function : Trigonometry
  Trigonometric Function1 : Trigonometry  Operator=cos
  f cos (rad) : Outport  VectorParamsAs1DForOutWhenUnconnected=off
  wires:
  Sum/1 -> Poduct/1, Poduct1/1
  Poduct/1 -> Kp/1
  Kp/1 -> Kp1/1
  Poduct2/1 -> Sum/2
  Trigonometric Function1/1 -> Poduct1/2, Poduct2/1
  Poduct1/1 -> K/1
  K/1 -> Integrator2/1
  Integrator2/1 -> Poduct2/2
  Integrator/1 -> Trigonometric Function/1, Sum2/2, Trigonometric Function1/1
  Integrator1/1 -> Sum2/1
  Sum2/1 -> f cos (rad)/1
  w/1 -> Sum1/1, Integrator1/1
  Kp1/1 -> Sum1/2
  Sum1/1 -> Integrator/1
  Trigonometric Function/1 -> Gain/1
  Gain/1 -> Poduct/2
  señal/1 -> Sum/1

== system Model_14Bus_AC_DC_Microgrid/Bus_AC//DC5/PLL/Pll2 ==
  note: error
  note: d'
  note: Fundamental
  note: fase
      | total
  note: fase de la señal
  note: adelanta 90
  note: Este PLL calcula la fase respecto a una onda coseno
  señal : Inport
  w : Inport  Port=2
  Gain : Gain  Gain=-1  SaturateOnIntegerOverflow=on  OutDataTypeStr=Inherit: Same as input  ParamDataTypeStr=Inherit: Same as input
  Integrator : Integrator  InitialCondition=2*pi*60
  Integrator1 : Integrator  InitialCondition=2*pi*60
  Integrator2 : Integrator
  K : Gain  Gain=100  SaturateOnIntegerOverflow=on  OutDataTypeStr=Inherit: Same as input  ParamDataTypeStr=Inherit: Same as input
  Kp : Gain  Gain=10  SaturateOnIntegerOverflow=on  OutDataTypeStr=Inherit: Same as input  ParamDataTypeStr=Inherit: Same as input
  Kp1 : Gain  Gain=10  SaturateOnIntegerOverflow=on  OutDataTypeStr=Inherit: Same as input  ParamDataTypeStr=Inherit: Same as input
  Poduct : Product  SaturateOnIntegerOverflow=on  OutDataTypeStr=Inherit: Same as first input
  Poduct1 : Product  SaturateOnIntegerOverflow=on  OutDataTypeStr=Inherit: Same as first input
  Poduct2 : Product  SaturateOnIntegerOverflow=on  OutDataTypeStr=Inherit: Same as first input
  Sum : Sum  Inputs=|+-  SaturateOnIntegerOverflow=on
  Sum1 : Sum  SaturateOnIntegerOverflow=on
  Sum2 : Sum  Inputs=|-+  SaturateOnIntegerOverflow=on
  Trigonometric Function : Trigonometry
  Trigonometric Function1 : Trigonometry  Operator=cos
  f cos (rad) : Outport  VectorParamsAs1DForOutWhenUnconnected=off
  wires:
  Sum/1 -> Poduct/1, Poduct1/1
  Poduct/1 -> Kp/1
  Kp/1 -> Kp1/1
  Poduct2/1 -> Sum/2
  Trigonometric Function1/1 -> Poduct1/2, Poduct2/1
  Poduct1/1 -> K/1
  K/1 -> Integrator2/1
  Integrator2/1 -> Poduct2/2
  Integrator/1 -> Trigonometric Function/1, Sum2/2, Trigonometric Function1/1
  Integrator1/1 -> Sum2/1
  Sum2/1 -> f cos (rad)/1
  w/1 -> Sum1/1, Integrator1/1
  Kp1/1 -> Sum1/2
  Sum1/1 -> Integrator/1
  Trigonometric Function/1 -> Gain/1
  Gain/1 -> Poduct/2
  señal/1 -> Sum/1

== system Model_14Bus_AC_DC_Microgrid/Bus_AC//DC5/PLL/Pll3 ==
  note: error
  note: d'
  note: Fundamental
  note: fase
      | total
  note: fase de la señal
  note: adelanta 90
  note: Este PLL calcula la fase respecto a una onda coseno
  señal : Inport
  w : Inport  Port=2
  Gain : Gain  Gain=-1  SaturateOnIntegerOverflow=on  OutDataTypeStr=Inherit: Same as input  ParamDataTypeStr=Inherit: Same as input
  Integrator : Integrator  InitialCondition=2*pi*60
  Integrator1 : Integrator  InitialCondition=2*pi*60
  Integrator2 : Integrator
  K : Gain  Gain=100  SaturateOnIntegerOverflow=on  OutDataTypeStr=Inherit: Same as input  ParamDataTypeStr=Inherit: Same as input
  Kp : Gain  Gain=10  SaturateOnIntegerOverflow=on  OutDataTypeStr=Inherit: Same as input  ParamDataTypeStr=Inherit: Same as input
  Kp1 : Gain  Gain=10  SaturateOnIntegerOverflow=on  OutDataTypeStr=Inherit: Same as input  ParamDataTypeStr=Inherit: Same as input
  Poduct : Product  SaturateOnIntegerOverflow=on  OutDataTypeStr=Inherit: Same as first input
  Poduct1 : Product  SaturateOnIntegerOverflow=on  OutDataTypeStr=Inherit: Same as first input
  Poduct2 : Product  SaturateOnIntegerOverflow=on  OutDataTypeStr=Inherit: Same as first input
  Sum : Sum  Inputs=|+-  SaturateOnIntegerOverflow=on
  Sum1 : Sum  SaturateOnIntegerOverflow=on
  Sum2 : Sum  Inputs=|-+  SaturateOnIntegerOverflow=on
  Trigonometric Function : Trigonometry
  Trigonometric Function1 : Trigonometry  Operator=cos
  f cos (rad) : Outport  VectorParamsAs1DForOutWhenUnconnected=off
  wires:
  Sum/1 -> Poduct/1, Poduct1/1
  Poduct/1 -> Kp/1
  Kp/1 -> Kp1/1
  Poduct2/1 -> Sum/2
  Trigonometric Function1/1 -> Poduct1/2, Poduct2/1
  Poduct1/1 -> K/1
  K/1 -> Integrator2/1
  Integrator2/1 -> Poduct2/2
  Integrator/1 -> Trigonometric Function/1, Sum2/2, Trigonometric Function1/1
  Integrator1/1 -> Sum2/1
  Sum2/1 -> f cos (rad)/1
  w/1 -> Sum1/1, Integrator1/1
  Kp1/1 -> Sum1/2
  Sum1/1 -> Integrator/1
  Trigonometric Function/1 -> Gain/1
  Gain/1 -> Poduct/2
  señal/1 -> Sum/1

== system Model_14Bus_AC_DC_Microgrid/Bus_slack /PLL/Pll1 ==
  note: error
  note: d'
  note: Fundamental
  note: fase
      | total
  note: fase de la señal
  note: adelanta 90
  note: Este PLL calcula la fase respecto a una onda coseno
  señal : Inport
  w : Inport  Port=2
  Gain : Gain  Gain=-1  SaturateOnIntegerOverflow=on  OutDataTypeStr=Inherit: Same as input  ParamDataTypeStr=Inherit: Same as input
  Integrator : Integrator  InitialCondition=2*pi*60
  Integrator1 : Integrator  InitialCondition=2*pi*60
  Integrator2 : Integrator
  K : Gain  Gain=100  SaturateOnIntegerOverflow=on  OutDataTypeStr=Inherit: Same as input  ParamDataTypeStr=Inherit: Same as input
  Kp : Gain  Gain=10  SaturateOnIntegerOverflow=on  OutDataTypeStr=Inherit: Same as input  ParamDataTypeStr=Inherit: Same as input
  Kp1 : Gain  Gain=10  SaturateOnIntegerOverflow=on  OutDataTypeStr=Inherit: Same as input  ParamDataTypeStr=Inherit: Same as input
  Poduct : Product  SaturateOnIntegerOverflow=on  OutDataTypeStr=Inherit: Same as first input
  Poduct1 : Product  SaturateOnIntegerOverflow=on  OutDataTypeStr=Inherit: Same as first input
  Poduct2 : Product  SaturateOnIntegerOverflow=on  OutDataTypeStr=Inherit: Same as first input
  Sum : Sum  Inputs=|+-  SaturateOnIntegerOverflow=on
  Sum1 : Sum  SaturateOnIntegerOverflow=on
  Sum2 : Sum  Inputs=|-+  SaturateOnIntegerOverflow=on
  Trigonometric Function : Trigonometry
  Trigonometric Function1 : Trigonometry  Operator=cos
  f cos (rad) : Outport  VectorParamsAs1DForOutWhenUnconnected=off
  wires:
  Sum/1 -> Poduct/1, Poduct1/1
  Poduct/1 -> Kp/1
  Kp/1 -> Kp1/1
  Poduct2/1 -> Sum/2
  Trigonometric Function1/1 -> Poduct1/2, Poduct2/1
  Poduct1/1 -> K/1
  K/1 -> Integrator2/1
  Integrator2/1 -> Poduct2/2
  Integrator/1 -> Trigonometric Function/1, Sum2/2, Trigonometric Function1/1
  Integrator1/1 -> Sum2/1
  Sum2/1 -> f cos (rad)/1
  w/1 -> Sum1/1, Integrator1/1
  Kp1/1 -> Sum1/2
  Sum1/1 -> Integrator/1
  Trigonometric Function/1 -> Gain/1
  Gain/1 -> Poduct/2
  señal/1 -> Sum/1

== system Model_14Bus_AC_DC_Microgrid/Bus_slack /PLL/Pll2 ==
  note: error
  note: d'
  note: Fundamental
  note: fase
      | total
  note: fase de la señal
  note: adelanta 90
  note: Este PLL calcula la fase respecto a una onda coseno
  señal : Inport
  w : Inport  Port=2
  Gain : Gain  Gain=-1  SaturateOnIntegerOverflow=on  OutDataTypeStr=Inherit: Same as input  ParamDataTypeStr=Inherit: Same as input
  Integrator : Integrator  InitialCondition=2*pi*60
  Integrator1 : Integrator  InitialCondition=2*pi*60
  Integrator2 : Integrator
  K : Gain  Gain=100  SaturateOnIntegerOverflow=on  OutDataTypeStr=Inherit: Same as input  ParamDataTypeStr=Inherit: Same as input
  Kp : Gain  Gain=10  SaturateOnIntegerOverflow=on  OutDataTypeStr=Inherit: Same as input  ParamDataTypeStr=Inherit: Same as input
  Kp1 : Gain  Gain=10  SaturateOnIntegerOverflow=on  OutDataTypeStr=Inherit: Same as input  ParamDataTypeStr=Inherit: Same as input
  Poduct : Product  SaturateOnIntegerOverflow=on  OutDataTypeStr=Inherit: Same as first input
  Poduct1 : Product  SaturateOnIntegerOverflow=on  OutDataTypeStr=Inherit: Same as first input
  Poduct2 : Product  SaturateOnIntegerOverflow=on  OutDataTypeStr=Inherit: Same as first input
  Sum : Sum  Inputs=|+-  SaturateOnIntegerOverflow=on
  Sum1 : Sum  SaturateOnIntegerOverflow=on
  Sum2 : Sum  Inputs=|-+  SaturateOnIntegerOverflow=on
  Trigonometric Function : Trigonometry
  Trigonometric Function1 : Trigonometry  Operator=cos
  f cos (rad) : Outport  VectorParamsAs1DForOutWhenUnconnected=off
  wires:
  Sum/1 -> Poduct/1, Poduct1/1
  Poduct/1 -> Kp/1
  Kp/1 -> Kp1/1
  Poduct2/1 -> Sum/2
  Trigonometric Function1/1 -> Poduct1/2, Poduct2/1
  Poduct1/1 -> K/1
  K/1 -> Integrator2/1
  Integrator2/1 -> Poduct2/2
  Integrator/1 -> Trigonometric Function/1, Sum2/2, Trigonometric Function1/1
  Integrator1/1 -> Sum2/1
  Sum2/1 -> f cos (rad)/1
  w/1 -> Sum1/1, Integrator1/1
  Kp1/1 -> Sum1/2
  Sum1/1 -> Integrator/1
  Trigonometric Function/1 -> Gain/1
  Gain/1 -> Poduct/2
  señal/1 -> Sum/1

== system Model_14Bus_AC_DC_Microgrid/Bus_slack /PLL/Pll3 ==
  note: error
  note: d'
  note: Fundamental
  note: fase
      | total
  note: fase de la señal
  note: adelanta 90
  note: Este PLL calcula la fase respecto a una onda coseno
  señal : Inport
  w : Inport  Port=2
  Gain : Gain  Gain=-1  SaturateOnIntegerOverflow=on  OutDataTypeStr=Inherit: Same as input  ParamDataTypeStr=Inherit: Same as input
  Integrator : Integrator  InitialCondition=2*pi*60
  Integrator1 : Integrator  InitialCondition=2*pi*60
  Integrator2 : Integrator
  K : Gain  Gain=100  SaturateOnIntegerOverflow=on  OutDataTypeStr=Inherit: Same as input  ParamDataTypeStr=Inherit: Same as input
  Kp : Gain  Gain=10  SaturateOnIntegerOverflow=on  OutDataTypeStr=Inherit: Same as input  ParamDataTypeStr=Inherit: Same as input
  Kp1 : Gain  Gain=10  SaturateOnIntegerOverflow=on  OutDataTypeStr=Inherit: Same as input  ParamDataTypeStr=Inherit: Same as input
  Poduct : Product  SaturateOnIntegerOverflow=on  OutDataTypeStr=Inherit: Same as first input
  Poduct1 : Product  SaturateOnIntegerOverflow=on  OutDataTypeStr=Inherit: Same as first input
  Poduct2 : Product  SaturateOnIntegerOverflow=on  OutDataTypeStr=Inherit: Same as first input
  Sum : Sum  Inputs=|+-  SaturateOnIntegerOverflow=on
  Sum1 : Sum  SaturateOnIntegerOverflow=on
  Sum2 : Sum  Inputs=|-+  SaturateOnIntegerOverflow=on
  Trigonometric Function : Trigonometry
  Trigonometric Function1 : Trigonometry  Operator=cos
  f cos (rad) : Outport  VectorParamsAs1DForOutWhenUnconnected=off
  wires:
  Sum/1 -> Poduct/1, Poduct1/1
  Poduct/1 -> Kp/1
  Kp/1 -> Kp1/1
  Poduct2/1 -> Sum/2
  Trigonometric Function1/1 -> Poduct1/2, Poduct2/1
  Poduct1/1 -> K/1
  K/1 -> Integrator2/1
  Integrator2/1 -> Poduct2/2
  Integrator/1 -> Trigonometric Function/1, Sum2/2, Trigonometric Function1/1
  Integrator1/1 -> Sum2/1
  Sum2/1 -> f cos (rad)/1
  w/1 -> Sum1/1, Integrator1/1
  Kp1/1 -> Sum1/2
  Sum1/1 -> Integrator/1
  Trigonometric Function/1 -> Gain/1
  Gain/1 -> Poduct/2
  señal/1 -> Sum/1
